simulink model "sampleModel324"  (R2021b)
settings: Solver=VariableStepAuto  StartTime=0.0  StopTime=10.0  RelTol=1e-3
undefined symbols (not defined in the file or in its folder): DiscIntNeverNeededParam, Newton, Raphson
libraries: simulink x8, slpidlib x2
settings Model: Creator=user  LastModifiedBy=user

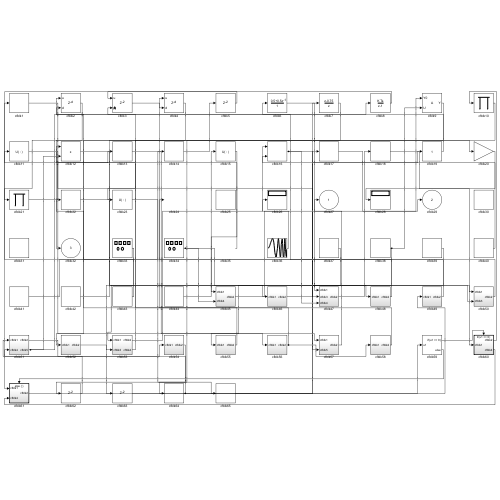
[thumbnail: Simulink's stored preview of the top-level diagram]
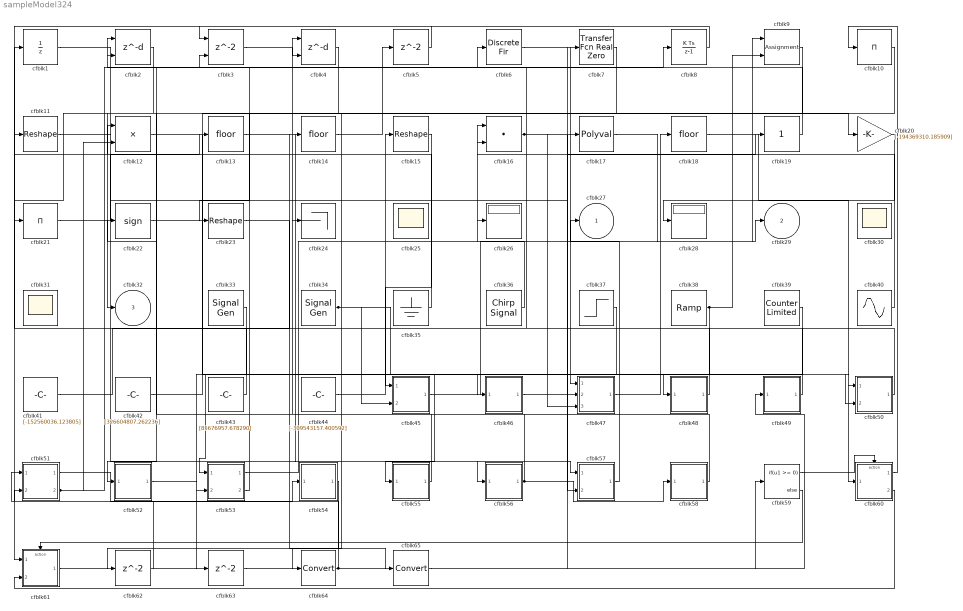
== system sampleModel324 ==
  cfblk1 : UnitDelay  HasFrameUpgradeWarning=on
  cfblk10 : Product  Inputs=*
  cfblk11 : Reshape
  cfblk12 : Product
  cfblk13 : Rounding
  cfblk14 : Rounding
  cfblk15 : Reshape
  cfblk16 : DotProduct  InputSameDT=on  OutDataTypeStr=Inherit: Inherit via internal rule
  cfblk17 : Polyval  Coefs=[ +2.081618890e-019, -1.441693666e-014, +4.719686976e-010, -8.536869453e-006, +1.621573104e-001, -8.087801117e+001 ]
  cfblk18 : Rounding
  cfblk19 : simulink/Math Operations/Slider Gain  gain=1  low=0  high=2
  cfblk2 : Delay  DelayLengthSource=Input port  SampleTime=1
      settings: InputPortMap=u0,p1
  cfblk20 : Gain  Gain=[-194369310.185909]
  cfblk21 : Product  Inputs=*
  cfblk22 : Signum
  cfblk23 : Reshape
  cfblk24 : Terminator
  cfblk25 : Scope
      settings: Floating=on
  cfblk26 : Display
  cfblk28 : Display
  cfblk3 : Delay  ShowEnablePort=on  SampleTime=1
      settings: InputPortMap=u0,e6
  cfblk30 : Scope
      settings: Floating=on
  cfblk31 : Scope
      settings: Floating=on
  cfblk33 : SignalGenerator  Amplitude=[-260960833.965020]
  cfblk34 : SignalGenerator  Amplitude=[93146175.689932]  Units=rad/sec
  cfblk35 : Ground
  cfblk36 : simulink/Sources/Chirp Signal  f1=[724895280.389638]  T=[171910445.014493]  f2=[778162531.520562]
  cfblk37 : Step  Time=[3.000000]  Before=[236796425.485370]  After=[-303609445.396841]  SampleTime=0
  cfblk38 : simulink/Sources/Ramp  slope=[-8175.117789]  start=[14.958853]  InitialOutput=[-371126.456777]
  cfblk39 : simulink/Sources/Counter Limited  uplimit=[293.000000]  tsamp=-1
  cfblk4 : Delay  DelayLengthSource=Input port  SampleTime=1
      settings: InputPortMap=u0,p1
  cfblk40 : Sin  Amplitude=[-801014828.780997]  Bias=[-914835470.871516]  SampleTime=0
  cfblk41 : Constant  Value=[-152560036.123805]  SampleTime=1
  cfblk42 : Constant  Value=[326604807.262236]  SampleTime=1
  cfblk43 : Constant  Value=[85676957.678290]  SampleTime=1
  cfblk44 : Constant  Value=[-309543157.400592]  SampleTime=1
  cfblk45 : Subsystem
  cfblk46 : Subsystem
  cfblk47 : Subsystem
  cfblk48 : Subsystem
  cfblk49 : Subsystem
  cfblk5 : Delay  SampleTime=1
  cfblk50 : Subsystem
  cfblk51 : Subsystem
  cfblk52 : Subsystem
  cfblk53 : Subsystem
  cfblk54 : Subsystem
  cfblk55 : Subsystem
  cfblk56 : Subsystem
  cfblk57 : Subsystem
  cfblk58 : Subsystem
  cfblk59 : If  IfExpression=u1 >= 0  SampleTime=1
  cfblk6 : DiscreteFir  SampleTime=1
  cfblk60 : Subsystem  TreatAsAtomicUnit=on
  cfblk61 : Subsystem  TreatAsAtomicUnit=on
  cfblk62 : Delay  SampleTime=1
  cfblk63 : Delay  SampleTime=1
  cfblk64 : DataTypeConversion
  cfblk65 : DataTypeConversion
  cfblk7 : simulink/Discrete/Transfer Fcn Real Zero  ZeroZ=0.75  ICPrevInput=0.0  DoSatur=off
      settings: SourceProductBaseCode=SL
  cfblk8 : DiscreteIntegrator  ICPrevOutput=DiscIntNeverNeededParam  ICPrevScaledInput=DiscIntNeverNeededParam
  cfblk9 : Assignment  DiagnosticForDimensions=Warning  IndexOptions=Index vector (dialog)  Indices=1  OutputSizes=1
  cfblk27 : Outport
  cfblk29 : Outport  Port=2
  cfblk32 : Outport  Port=3
  wires:
  cfblk53/1(cfblk2) -> cfblk16/1
  cfblk13/1 -> cfblk56/1(cfblk1)
  cfblk42/1 -> cfblk20/1
  cfblk61/1(cfblk2) -> cfblk49/1(cfblk1)
  cfblk20/1 -> cfblk28/1
  cfblk6/1 -> cfblk47/1(cfblk1)
  cfblk8/1 -> cfblk61/1(cfblk1)
  cfblk55/1(cfblk2) -> cfblk4/1
  cfblk56/1(cfblk2) -> cfblk58/1(cfblk1), cfblk3/2
  cfblk50/1(cfblk2) -> cfblk24/1
  cfblk17/1 -> cfblk29/1
  cfblk33/1 -> cfblk53/1(cfblk1)
  cfblk12/1 -> cfblk48/1(cfblk1)
  cfblk21/1 -> cfblk13/1
  cfblk38/1 -> cfblk47/2(cfblk3), cfblk9/2
  cfblk1/1 -> cfblk57/1(cfblk1)
  cfblk47/1(cfblk2) -> cfblk18/1
  cfblk3/1 -> cfblk4/2
  cfblk18/1 -> cfblk60/1(cfblk1)
  cfblk40/1 -> cfblk16/2
  cfblk2/1 -> cfblk32/1
  cfblk44/1 -> cfblk15/1
  cfblk51/1(cfblk2) -> cfblk54/1(cfblk1)
  cfblk7/1 -> cfblk64/1
  cfblk10/1 -> cfblk52/1(cfblk1)
  cfblk15/1 -> cfblk45/1(cfblk1)
  cfblk14/1 -> cfblk5/1
  cfblk49/1(cfblk2) -> cfblk1/1
  cfblk58/1(cfblk2) -> cfblk22/1
  cfblk60/1(cfblk2) -> cfblk10/1
  cfblk11/1 -> cfblk57/2(cfblk5)
  cfblk53/2(cfblk4) -> cfblk11/1
  cfblk36/1 -> cfblk26/1
  cfblk45/1(cfblk2) -> cfblk9/1
  cfblk5/1 -> cfblk3/1
  cfblk39/1 -> cfblk55/1(cfblk1)
  cfblk43/1 -> cfblk12/1
  cfblk19/1 -> cfblk2/1
  cfblk60/2(cfblk4) -> cfblk61/2(cfblk4)
  cfblk22/1 -> cfblk46/1(cfblk1)
  cfblk48/1(cfblk2) -> cfblk6/1
  cfblk37/1 -> cfblk53/2(cfblk3)
  cfblk57/1(cfblk2) -> cfblk27/1
  cfblk51/2(cfblk5) -> cfblk8/1, cfblk12/2
  cfblk16/1 -> cfblk50/1(cfblk1), cfblk47/3(cfblk4)
  cfblk9/1 -> cfblk21/1
  cfblk34/1 -> cfblk50/2(cfblk3), cfblk45/2(cfblk4)
  cfblk35/1 -> cfblk2/2
  cfblk41/1 -> cfblk14/1
  cfblk4/1 -> cfblk23/1
  cfblk46/1(cfblk2) -> cfblk19/1
  cfblk59/1 -> cfblk60/Action
  cfblk59/2 -> cfblk61/Action
  cfblk54/1(cfblk2) -> cfblk62/1
  cfblk62/1 -> cfblk51/1(cfblk1)
  cfblk52/1(cfblk2) -> cfblk63/1
  cfblk63/1 -> cfblk59/1
  cfblk64/1 -> cfblk51/2(cfblk4), cfblk17/1
  cfblk23/1 -> cfblk65/1
  cfblk65/1 -> cfblk7/1

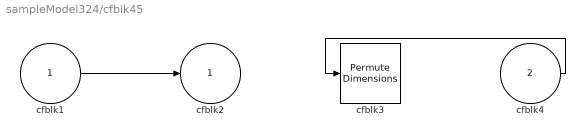
== system sampleModel324/cfblk45 ==
  cfblk1 : Inport
  cfblk4 : Inport  Port=2
  cfblk3 : PermuteDimensions
  cfblk2 : Outport
  wires:
  cfblk1/1 -> cfblk2/1
  cfblk4/1 -> cfblk3/1

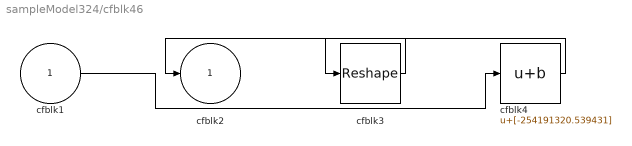
== system sampleModel324/cfblk46 ==
  cfblk1 : Inport
  cfblk3 : Reshape
  cfblk4 : Bias  Bias=[-254191320.539431]
  cfblk2 : Outport
  wires:
  cfblk3/1 -> cfblk2/1
  cfblk1/1 -> cfblk4/1
  cfblk4/1 -> cfblk3/1

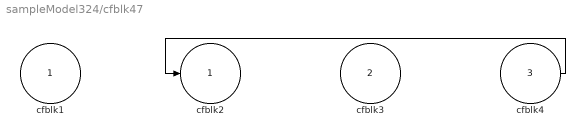
== system sampleModel324/cfblk47 ==
  cfblk1 : Inport
  cfblk3 : Inport  Port=2
  cfblk4 : Inport  Port=3
  cfblk2 : Outport
  wires:
  cfblk4/1 -> cfblk2/1

== system sampleModel324/cfblk48 ==
  cfblk1 : Inport
  cfblk3 : Delay  SampleTime=1
  cfblk2 : Outport
  wires:
  cfblk1/1 -> cfblk3/1
  cfblk3/1 -> cfblk2/1

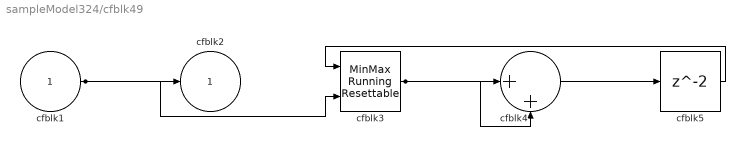
== system sampleModel324/cfblk49 ==
  cfblk1 : Inport
  cfblk3 : simulink/Math Operations/MinMax Running Resettable  Function=min  vinit=0.0
  cfblk4 : Sum  Inputs=|++
  cfblk5 : Delay  SampleTime=1
  cfblk2 : Outport
  wires:
  cfblk1/1 -> cfblk2/1, cfblk3/2
  cfblk3/1 -> cfblk4/1, cfblk4/2
  cfblk4/1 -> cfblk5/1
  cfblk5/1 -> cfblk3/1

== system sampleModel324/cfblk50 ==
  cfblk1 : Inport
  cfblk3 : Inport  Port=2
  cfblk2 : Outport
  wires:
  cfblk3/1 -> cfblk2/1

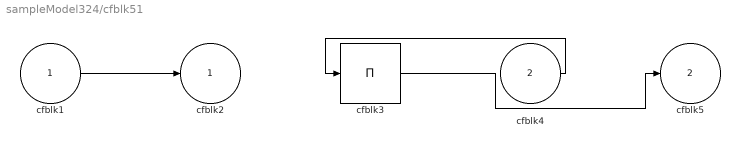
== system sampleModel324/cfblk51 ==
  cfblk1 : Inport
  cfblk4 : Inport  Port=2
  cfblk3 : Product  Inputs=*
  cfblk2 : Outport
  cfblk5 : Outport  Port=2
  wires:
  cfblk1/1 -> cfblk2/1
  cfblk4/1 -> cfblk3/1
  cfblk3/1 -> cfblk5/1

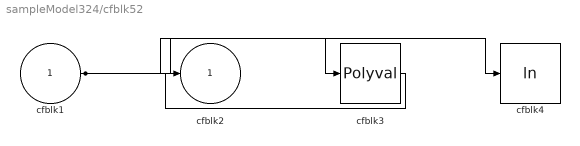
== system sampleModel324/cfblk52 ==
  cfblk1 : Inport
  cfblk3 : Polyval  Coefs=[ +2.081618890e-019, -1.441693666e-014, +4.719686976e-010, -8.536869453e-006, +1.621573104e-001, -8.087801117e+001 ]
  cfblk4 : Math  Operator=log  SaturateOnIntegerOverflow=on
  cfblk2 : Outport
  wires:
  cfblk1/1 -> cfblk3/1, cfblk4/1
  cfblk3/1 -> cfblk2/1

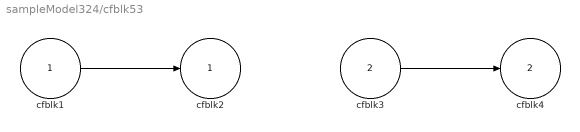
== system sampleModel324/cfblk53 ==
  cfblk1 : Inport
  cfblk3 : Inport  Port=2
  cfblk2 : Outport
  cfblk4 : Outport  Port=2
  wires:
  cfblk3/1 -> cfblk4/1
  cfblk1/1 -> cfblk2/1

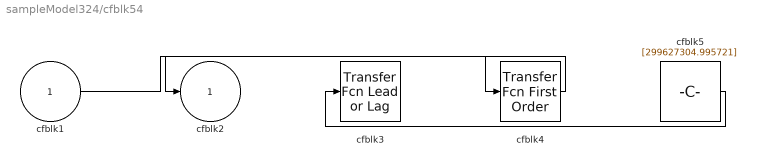
== system sampleModel324/cfblk54 ==
  cfblk1 : Inport
  cfblk3 : simulink/Discrete/Transfer Fcn Lead or Lag  PoleZ=0.95  ZeroZ=0.75  ICPrevOutput=0.0  ICPrevInput=0.0  DoSatur=off
      settings: SourceProductBaseCode=SL
  cfblk4 : simulink/Discrete/Transfer Fcn First Order  PoleZ=0.95  ICPrevOutput=0.0  DoSatur=off
  cfblk5 : Constant  Value=[299627304.995721]  SampleTime=1
  cfblk2 : Outport
  wires:
  cfblk4/1 -> cfblk2/1
  cfblk5/1 -> cfblk3/1
  cfblk1/1 -> cfblk4/1

== system sampleModel324/cfblk55 ==
  cfblk1 : Inport
  cfblk3 : Constant  Value=[659463096.950788]  SampleTime=1
  cfblk2 : Outport
  wires:
  cfblk1/1 -> cfblk2/1

== system sampleModel324/cfblk56 ==
  cfblk1 : Inport
  cfblk3 : DiscreteIntegrator  ICPrevOutput=DiscIntNeverNeededParam  ICPrevScaledInput=DiscIntNeverNeededParam
  cfblk4 : slpidlib/PID Controller  Controller=PID  Form=Parallel  TimeDomain=Discrete-time  UseExternalTs=off  SampleTime=1  IntegratorMethod=Forward Euler  FilterMethod=Forward Euler  ControllerParametersSource=internal  P=1  I=1  D=0  UseFilter=on  N=100  TunerSelectOption=Transfer Function Based (PID Tuner App)  InitialConditionSource=internal  InitialConditionForIntegrator=0  InitialConditionForFilter=0  DifferentiatorICPrevScaledInput=0  ExternalReset=none  TrackingMode=off  Kt=1  LimitOutput=off  SatLimitsSource=internal  UpperSaturationLimit=inf  LowerSaturationLimit=-inf  LinearizeAsGain=off  AntiWindupMode=none  Kb=1  POutMin=[]  POutMax=[]  IOutMin=[]  IOutMax=[]  DOutMin=[]  DOutMax=[]  NOutMin=[]  NOutMax=[]  SumOutMin=[]  SumOutMax=[]  SaturationOutMin=[]  SaturationOutMax=[]  PParamMin=[]  PParamMax=[]  IParamMin=[]  IParamMax=[]  DParamMin=[]  DParamMax=[]  NParamMin=[]  NParamMax=[]  KbParamMin=[]  KbParamMax=[]  KtParamMin=[]  KtParamMax=[]  KbOutMin=[]  KbOutMax=[]  KtOutMin=[]  KtOutMax=[]  IntegratorOutMin=[]  IntegratorOutMax=[]  FilterOutMin=[]  FilterOutMax=[]  SumI1OutMin=[]  SumI1OutMax=[]  SumI2OutMin=[]  SumI2OutMax=[]  SumI3OutMin=[]  SumI3OutMax=[]  SumI4OutMin=[]  SumI4OutMax=[]  SumDOutMin=[]  SumDOutMax=[]  DifferentiatorOutMin=[]  DifferentiatorOutMax=[]  FilterDiffOutCoefMin=[]  FilterDiffOutCoefMax=[]  ReciprocalOutMin=[]  ReciprocalOutMax=[]  SumDenOutMin=[]  SumDenOutMax=[]  SumNumOutMin=[]  SumNumOutMax=[]  DivideOutMin=[]  DivideOutMax=[]  UdiffTsProdOutMin=[]  UdiffTsProdOutMax=[]  NTsProdOutMin=[]  NTsProdOutMax=[]  UintegralTsProdOutMin=[]  UintegralTsProdOutMax=[]  UngainTsProdOutMin=[]  UngainTsProdOutMax=[]  IntegratorContinuousStateAttributes=''  IntegratorStateMustResolveToSignalObject=off  IntegratorRTWStateStorageClass=Auto  FilterContinuousStateAttributes=''  FilterStateMustResolveToSignalObject=off  FilterRTWStateStorageClass=Auto  ParallelPVariant=InternalParameters  IdealPVariant=Disabled  IVariant=InternalParameters  DVariant=InternalParameters  IntegratorVariant=Discrete  SatVariant=Disabled  AWVariant=Passthrough  PCopyVariant=Disabled  TRVariant=Disabled  FdbkBlocksVariant=Forward  IdealPFdbkVariant=Disabled  SatFdbkVariant=Disabled  DerivativeFilterVariant=ForwardEulerFilter  NVariant=InternalParameters  NCopyVariant=Disabled  FilterICVariant=InternalICsFilter  IntegratorICVariant=InternalICs  ExternalResetVariant=Disabled  TRSumVariant=Passthrough  SumFdbkVariant=Disabled  SumVariant=Sum_PID  TsampFilterVariant=InternalTs  TsampNgainVariant=Passthrough  TsampIntegralVariant=Passthrough  ExternalSaturationOutDataTypeStr=Inherit: Same as second input
  cfblk2 : Outport
  wires:
  cfblk1/1 -> cfblk4/1
  cfblk4/1 -> cfblk3/1
  cfblk3/1 -> cfblk2/1

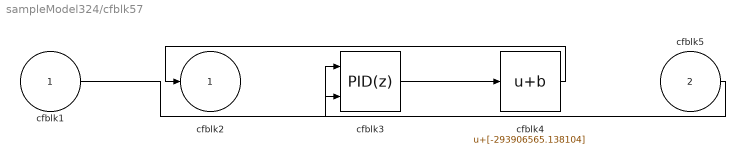
== system sampleModel324/cfblk57 ==
  cfblk1 : Inport
  cfblk5 : Inport  Port=2
  cfblk3 : slpidlib/PID Controller (2DOF)  Controller=PID  Form=Parallel  TimeDomain=Discrete-time  UseExternalTs=off  SampleTime=1  IntegratorMethod=Forward Euler  FilterMethod=Forward Euler  ControllerParametersSource=internal  P=1  I=1  D=0  UseFilter=on  N=100  b=1  c=1  TunerSelectOption=Transfer Function Based (PID Tuner App)  InitialConditionSource=internal  InitialConditionForIntegrator=0  InitialConditionForFilter=0  DifferentiatorICPrevScaledInput=0  ExternalReset=none  TrackingMode=off  Kt=1  LimitOutput=off  SatLimitsSource=internal  UpperSaturationLimit=inf  LowerSaturationLimit=-inf  LinearizeAsGain=off  AntiWindupMode=none  Kb=1  POutMin=[]  POutMax=[]  IOutMin=[]  IOutMax=[]  DOutMin=[]  DOutMax=[]  NOutMin=[]  NOutMax=[]  bOutMin=[]  bOutMax=[]  cOutMin=[]  cOutMax=[]  SumOutMin=[]  SumOutMax=[]  SaturationOutMin=[]  SaturationOutMax=[]  PParamMin=[]  PParamMax=[]  IParamMin=[]  IParamMax=[]  DParamMin=[]  DParamMax=[]  NParamMin=[]  NParamMax=[]  bParamMin=[]  bParamMax=[]  cParamMin=[]  cParamMax=[]  KbParamMin=[]  KbParamMax=[]  KtParamMin=[]  KtParamMax=[]  KbOutMin=[]  KbOutMax=[]  KtOutMin=[]  KtOutMax=[]  IntegratorOutMin=[]  IntegratorOutMax=[]  FilterOutMin=[]  FilterOutMax=[]  SumI1OutMin=[]  SumI1OutMax=[]  SumI2OutMin=[]  SumI2OutMax=[]  SumI3OutMin=[]  SumI3OutMax=[]  SumI4OutMin=[]  SumI4OutMax=[]  SumDOutMin=[]  SumDOutMax=[]  Sum1OutMin=[]  Sum1OutMax=[]  Sum2OutMin=[]  Sum2OutMax=[]  Sum3OutMin=[]  Sum3OutMax=[]  DifferentiatorOutMin=[]  DifferentiatorOutMax=[]  FilterDiffOutCoefMin=[]  FilterDiffOutCoefMax=[]  ReciprocalOutMin=[]  ReciprocalOutMax=[]  SumDenOutMin=[]  SumDenOutMax=[]  SumNumOutMin=[]  SumNumOutMax=[]  DivideOutMin=[]  DivideOutMax=[]  UdiffTsProdOutMin=[]  UdiffTsProdOutMax=[]  NTsProdOutMin=[]  NTsProdOutMax=[]  UintegralTsProdOutMin=[]  UintegralTsProdOutMax=[]  UngainTsProdOutMin=[]  UngainTsProdOutMax=[]  IntegratorContinuousStateAttributes=''  IntegratorStateMustResolveToSignalObject=off  IntegratorRTWStateStorageClass=Auto  FilterContinuousStateAttributes=''  FilterStateMustResolveToSignalObject=off  FilterRTWStateStorageClass=Auto  ParallelPVariant=InternalParameters  IdealPVariant=Disabled  IVariant=InternalParameters  DVariant=InternalParameters  bVariant=InternalParameters  cVariant=InternalParameters  IntegratorVariant=Discrete  SatVariant=Disabled  AWVariant=Passthrough  PCopyVariant=Disabled  TRVariant=Disabled  FdbkBlocksVariant=Forward  IdealPFdbkVariant=Disabled  SatFdbkVariant=Disabled  DerivativeFilterVariant=ForwardEulerFilter  NVariant=InternalParameters  NCopyVariant=Disabled  FilterICVariant=InternalICsFilter  IntegratorICVariant=InternalICs  ExternalResetVariant=Disabled  TRSumVariant=Passthrough  SumFdbkVariant=Disabled  SumVariant=Sum_PID  TsampFilterVariant=InternalTs  TsampNgainVariant=Passthrough  TsampIntegralVariant=Passthrough  ExternalSaturationOutDataTypeStr=Inherit: Same as second input
      settings: SourceProductBaseCode=SL
  cfblk4 : Bias  Bias=[-293906565.138104]
  cfblk2 : Outport
  wires:
  cfblk3/1 -> cfblk4/1
  cfblk4/1 -> cfblk2/1
  cfblk5/1 -> cfblk3/1
  cfblk1/1 -> cfblk3/2

== system sampleModel324/cfblk58 ==
  cfblk1 : Inport
  cfblk3 : Constant  Value=[-301300954.411194]  SampleTime=1
  cfblk2 : Outport
  wires:
  cfblk3/1 -> cfblk2/1

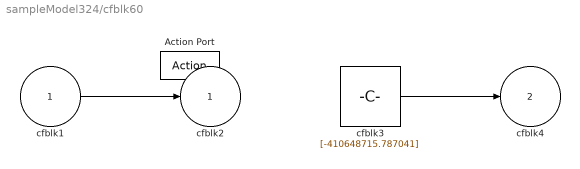
== system sampleModel324/cfblk60 ==
  cfblk1 : Inport
  Action Port : ActionPort  ActionPortLabel=if(u1 >= 0)
  cfblk3 : Constant  Value=[-410648715.787041]  SampleTime=1
  cfblk2 : Outport
  cfblk4 : Outport  Port=2
  wires:
  cfblk1/1 -> cfblk2/1
  cfblk3/1 -> cfblk4/1

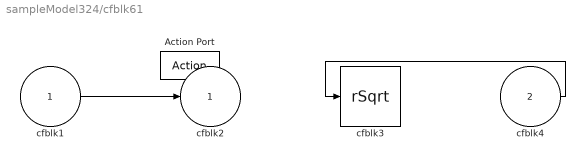
== system sampleModel324/cfblk61 ==
  cfblk1 : Inport
  cfblk4 : Inport  Port=2
  Action Port : ActionPort  ActionPortLabel=else
  cfblk3 : Sqrt  Operator=rSqrt  AlgorithmType=Newton-Raphson  SaturateOnIntegerOverflow=on
  cfblk2 : Outport
  wires:
  cfblk4/1 -> cfblk3/1
  cfblk1/1 -> cfblk2/1
